simulink subsystem "BaseDriver"  (R2020b)
settings: Solver=VariableStepAuto  StartTime=0.0  StopTime=10.0  RelTol=1e-3
undefined symbols (not defined in the file): maxAngles, maxOmega, ts_control
libraries: Library x7
settings Model: Creator=alons  LastModifiedBy=elbit

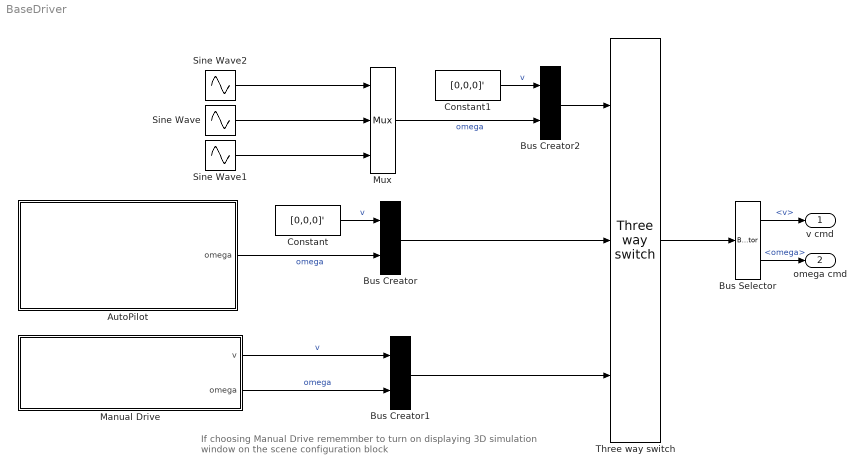
== system BaseDriver ==
  note: If choosing Manual Drive rememmber to turn on displaying 3D simulation window on the scene configuration block
  AutoPilot : Subsystem  mask{Tswitch=3, roll_vlim=maxOmega(1)*[0,1], roll_xlim=maxAngles(1)*[-1,1], pitch_vlim=eps*maxOmega(2)*[0,1], pitch_xlim=maxAngles(2)*[-1,1], yaw_vlim=eps*maxOmega(3)*[0,1], yaw_xlim=maxAngles(3)*[-1,1]}
      mask prompts: roll_vlim "abs vlim range[rad/s]"; roll_xlim "xlim range [rad]"; pitch_vlim "abs vlim range [rad/s]"; pitch_xlim "xlim range [rad]"; yaw_vlim "abs vlim range [rad/s]"; yaw_xlim "xlim range [rad]"
      mask init:
      | bounds=[roll_xlim;
      |     pitch_xlim;
      |     yaw_xlim];
      mask DialogControl roll_container Prompt: roll
      mask DialogControl pitch_container Prompt: pitch
      mask DialogControl yaw_container Prompt: yaw
  Bus Creator : BusCreator  Inputs=2
  Bus Creator1 : BusCreator  Inputs=2
  Bus Creator2 : BusCreator  Inputs=2
  Bus Selector : BusSelector  OutputSignals=v,omega
  Constant : Constant  Value=[0,0,0]'
  Constant1 : Constant  Value=[0,0,0]'
  Manual Drive : Subsystem
  Mux : Mux  Inputs=3
  Sine Wave : Sin  Amplitude=0*(6/10)*maxOmega(2)  Frequency=2*pi*0.5  Phase=pi/2  SampleTime=0
  Sine Wave1 : Sin  Amplitude=0*maxOmega(3)  Frequency=2*pi*1  Phase=pi/2  SampleTime=0
  Sine Wave2 : Sin  Amplitude=maxOmega(1)  Frequency=2*pi*1  Phase=pi/2  SampleTime=0
  Three way switch : Library/Basics/Three way switch  Choice=2
  v cmd : Outport
  omega cmd : Outport  Port=2
  wires:
  Constant/1 -> Bus Creator/1  "v"
  Bus Selector/2 -> omega cmd/1  "<omega>"
  Bus Selector/1 -> v cmd/1  "<v>"
  AutoPilot/1(omega) -> Bus Creator/2  "omega"
  Manual Drive/1(v) -> Bus Creator1/1  "v"
  Bus Creator/1 -> Three way switch/2
  Manual Drive/2(omega) -> Bus Creator1/2  "omega"
  Bus Creator1/1 -> Three way switch/3
  Mux/1 -> Bus Creator2/2  "omega"
  Constant1/1 -> Bus Creator2/1  "v"
  Sine Wave2/1 -> Mux/1
  Sine Wave1/1 -> Mux/3
  Sine Wave/1 -> Mux/2
  Bus Creator2/1 -> Three way switch/1
  Three way switch/1 -> Bus Selector/1

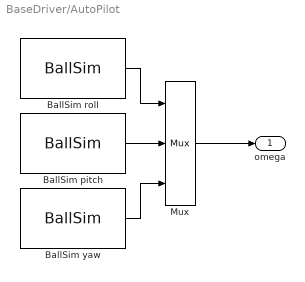
== system BaseDriver/AutoPilot ==
  BallSim pitch : Library/Event Camera/BallSim  vlim=pitch_vlim  xlim=pitch_xlim  Tswitch=Tswitch
  BallSim roll : Library/Event Camera/BallSim  vlim=roll_vlim  xlim=roll_xlim  Tswitch=Tswitch
  BallSim yaw : Library/Event Camera/BallSim  vlim=yaw_vlim  xlim=yaw_xlim  Tswitch=Tswitch
  Mux : Mux  Inputs=3
  omega : Outport
  wires:
  Mux/1 -> omega/1
  BallSim yaw/1 -> Mux/3
  BallSim roll/1 -> Mux/1
  BallSim pitch/1 -> Mux/2

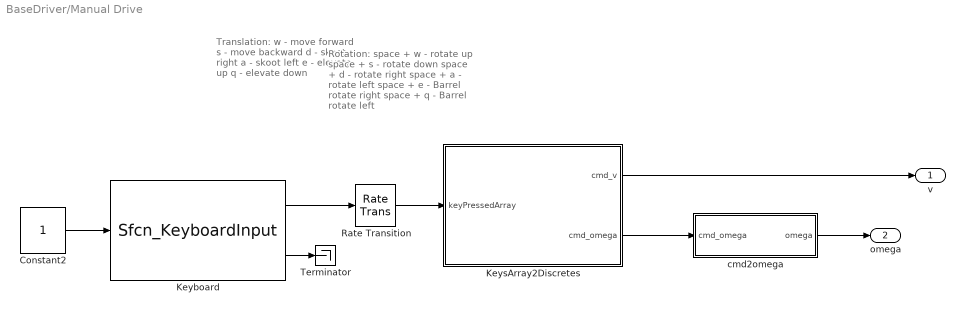
== system BaseDriver/Manual Drive ==
  note: Translation:
      | w - move forward
      | s - move backward
      | d - skoot right
      | a - skoot left
      | e - elevate up
      | q - elevate down
  note: Rotation:
      | space + w - rotate up
      | space + s - rotate down
      | space + d - rotate right
      | space + a - rotate left
      | space + e - Barrel rotate right
      | space + q - Barrel rotate left
  Constant2 : Constant
      settings: OpenFcn=|
      | if get_param(gcbh,'value')-48
      |    set_param(gcbh,'value','0','backgroundcolor','red');
      | else
      |    set_param(gcbh,'value','1','backgroundcolor','green');
      | end
  Keyboard : M-S-Function  FunctionName=Sfcn_KeyboardInput  Parameters=ts_control*100
  KeysArray2Discretes : MATLAB Function  TreatAsAtomicUnit=on
  Rate Transition : RateTransition
  Terminator : Terminator
  cmd2omega : Subsystem  TreatAsAtomicUnit=on
  v : Outport
  omega : Outport  Port=2
  wires:
  Keyboard/1 -> Rate Transition/1
  Rate Transition/1 -> KeysArray2Discretes/1(keyPressedArray)
  KeysArray2Discretes/1(cmd_v) -> v/1
  KeysArray2Discretes/2(cmd_omega) -> cmd2omega/1(cmd_omega)
  cmd2omega/1(omega) -> omega/1
  Keyboard/2 -> Terminator/1
  Constant2/1 -> Keyboard/1

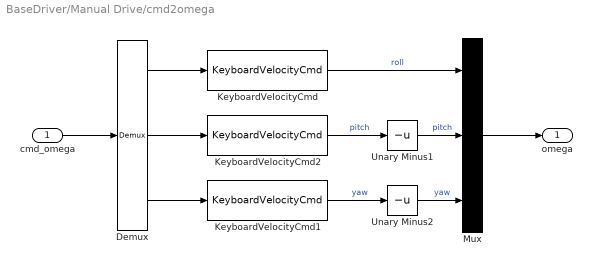
== system BaseDriver/Manual Drive/cmd2omega ==
  cmd_omega : Inport
  Demux : Demux  Outputs=3
  KeyboardVelocityCmd : Library/Event Camera/KeyboardVelocityCmd  max=maxOmega(1)  step_percentile=0.2
  KeyboardVelocityCmd1 : Library/Event Camera/KeyboardVelocityCmd  max=maxOmega(3)  step_percentile=0.2
  KeyboardVelocityCmd2 : Library/Event Camera/KeyboardVelocityCmd  max=maxOmega(2)  step_percentile=0.2
  Mux : Mux  Inputs=3
  Unary Minus1 : UnaryMinus
  Unary Minus2 : UnaryMinus
  omega : Outport
  wires:
  Unary Minus2/1 -> Mux/3  "yaw"
  Unary Minus1/1 -> Mux/2  "pitch"
  KeyboardVelocityCmd1/1 -> Unary Minus2/1  "yaw"
  KeyboardVelocityCmd2/1 -> Unary Minus1/1  "pitch"
  KeyboardVelocityCmd/1 -> Mux/1  "roll"
  Mux/1 -> omega/1
  Demux/1 -> KeyboardVelocityCmd/1
  Demux/2 -> KeyboardVelocityCmd2/1
  Demux/3 -> KeyboardVelocityCmd1/1
  cmd_omega/1 -> Demux/1

== matlab function BaseDriver/Manual Drive/KeysArray2Discretes ==
  data: keyPressedArray input; cmd_v output; cmd_omega output
function [cmd_v,cmd_omega] = KeysArray2Discretes(keyPressedArray)
spacePressed=keyPressedArray(1);

if spacePressed %Rotational movement
    up=keyPressedArray(2); %w
    down=keyPressedArray(3); %s
    right=keyPressedArray(4); %d
    left=keyPressedArray(5); %a
    rollRight=keyPressedArray(6); %e
    rollLeft=keyPressedArray(7); %q
    
    cmd_v=[0;0;0];
    cmd_omega=[rollRight-rollLeft %roll
        up-down; %pitch
        right-left]; %yaw
    
else %Translational movement
    forward=keyPressedArray(2); %w
    backward=keyPressedArray(3); %s
    right=keyPressedArray(4); %d
    left=keyPressedArray(5); %a
    up=keyPressedArray(6); %e
    down=keyPressedArray(7); %q
    
    cmd_omega=[0;0;0];
    cmd_v=[forward-backward;
        right-left;
        up-down];
end
